simulink model "power_limiter"  (R2024a)
settings: Solver=VariableStepAuto  StartTime=0.0  StopTime=10.0  RelTol=1e-3
values from neighbouring files (symbols this model uses):
  Ki_pl = 0.01    [srcipt.m]
  Kp_pl = 0.1    [srcipt.m]
  Ts = 0.01    [srcipt.m]
settings Model: Creator=DELL  LastModifiedBy=DELL

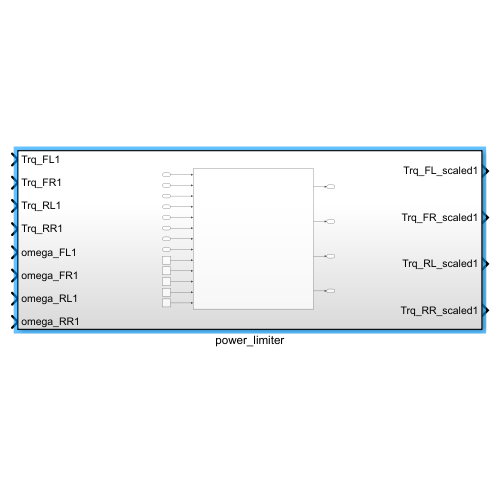
[thumbnail: Simulink's stored preview of the top-level diagram]
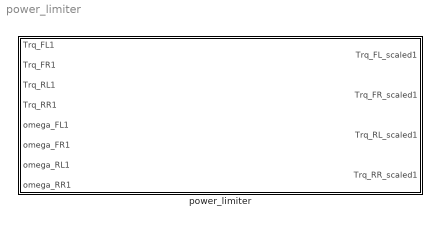
== system power_limiter ==
  power_limiter : Subsystem

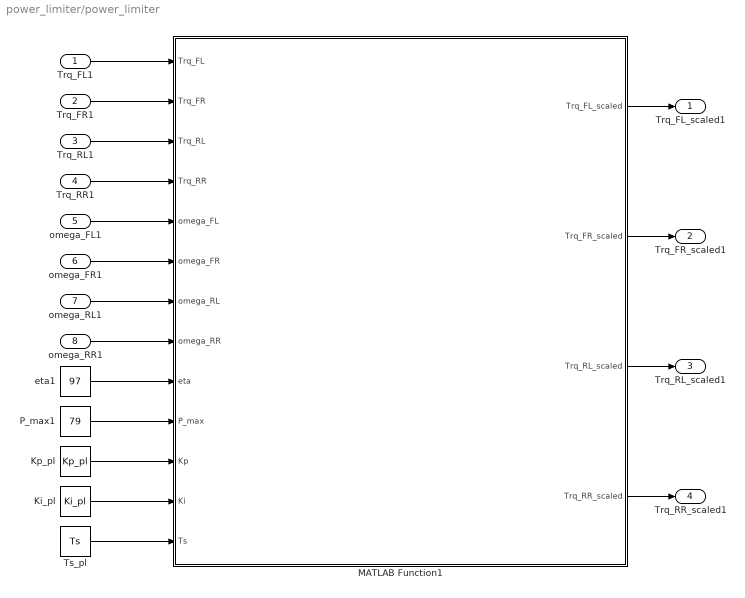
== system power_limiter/power_limiter ==
  Trq_FL1 : Inport
  Trq_FR1 : Inport  Port=2
  Trq_RL1 : Inport  Port=3
  Trq_RR1 : Inport  Port=4
  omega_FL1 : Inport  Port=5
  omega_FR1 : Inport  Port=6
  omega_RL1 : Inport  Port=7
  omega_RR1 : Inport  Port=8
  Ki_pl : Constant  Value=Ki_pl
  Kp_pl : Constant  Value=Kp_pl
  MATLAB Function1 : MATLAB Function  TreatAsAtomicUnit=on
  P_max1 : Constant  Value=79
  Ts_pl : Constant  Value=Ts
  eta1 : Constant  Value=97
  Trq_FL_scaled1 : Outport
  Trq_FR_scaled1 : Outport  Port=2
  Trq_RL_scaled1 : Outport  Port=3
  Trq_RR_scaled1 : Outport  Port=4
  wires:
  Kp_pl/1 -> MATLAB Function1/11(Kp)
  Trq_FL1/1 -> MATLAB Function1/1(Trq_FL)
  eta1/1 -> MATLAB Function1/9(eta)
  MATLAB Function1/3(Trq_RL_scaled) -> Trq_RL_scaled1/1
  MATLAB Function1/1(Trq_FL_scaled) -> Trq_FL_scaled1/1
  Ts_pl/1 -> MATLAB Function1/13(Ts)
  Ki_pl/1 -> MATLAB Function1/12(Ki)
  Trq_FR1/1 -> MATLAB Function1/2(Trq_FR)
  MATLAB Function1/4(Trq_RR_scaled) -> Trq_RR_scaled1/1
  Trq_RR1/1 -> MATLAB Function1/4(Trq_RR)
  omega_FL1/1 -> MATLAB Function1/5(omega_FL)
  P_max1/1 -> MATLAB Function1/10(P_max)
  omega_RL1/1 -> MATLAB Function1/7(omega_RL)
  MATLAB Function1/2(Trq_FR_scaled) -> Trq_FR_scaled1/1
  Trq_RL1/1 -> MATLAB Function1/3(Trq_RL)
  omega_RR1/1 -> MATLAB Function1/8(omega_RR)
  omega_FR1/1 -> MATLAB Function1/6(omega_FR)

== matlab function power_limiter/MATLAB Function1 ==
  settings: updateMethod=DISCRETE  sampleTime=Ts
  data: Trq_FL input; Trq_FL_scaled output; Trq_FR input; Trq_RL input; Trq_RR input; omega_FL input; omega_FR input; omega_RL input; omega_RR input; eta input; P_max input; Trq_FR_scaled output; Trq_RL_scaled output; Trq_RR_scaled output; Kp input; Ki input; Ts input
function [Trq_FL_scaled, Trq_FR_scaled, Trq_RL_scaled, Trq_RR_scaled] = ... 
    scaleTorqueToPowerLimit_PI(Trq_FL, Trq_FR, Trq_RL, Trq_RR, ... 
    omega_FL, omega_FR, omega_RL, omega_RR, eta, P_max, Kp, Ki, Ts)
    % Input parameters:
    % Trq_FL, Trq_FR, Trq_RL, Trq_RR - torque on each wheel
    % omega_FL, omega_FR, omega_RL, omega_RR - angular velocity of each wheel
    % eta - motor efficiency
    % P_max - maximum battery power = 79kW
    % Kp - proportional gain
    % Ki - integral gain
    % Ts - sampling time

    persistent integral_error;
    if isempty(integral_error)
        integral_error = 0;
    end

    P_mech_FL = Trq_FL * omega_FL;
    P_mech_FR = Trq_FR * omega_FR;
    P_mech_RL = Trq_RL * omega_RL;
    P_mech_RR = Trq_RR * omega_RR;
    
    P_mech_total = P_mech_FL + P_mech_FR + P_mech_RL + P_mech_RR;
    
    P_el_total = P_mech_total / eta;

    % PI controller
    error = P_max - P_el_total;
    integral_error = integral_error + error * Ts;
    control_signal = Kp * error + Ki * integral_error;


    if control_signal < 0
        scale_factor = 0;
    else
        scale_factor = min(1, control_signal);
    end
    
    Trq_FL_scaled = Trq_FL * scale_factor;
    Trq_FR_scaled = Trq_FR * scale_factor;
    Trq_RL_scaled = Trq_RL * scale_factor;
    Trq_RR_scaled = Trq_RR * scale_factor;
end
